simulink model "Airbrake_sim_newpso"  (R2023b)
settings: Solver=FixedStepAuto  StartTime=0.0  StopTime=30  FixedStep=0.01  RelTol=1e-3
model workspace (MAT data in the model file):
  surfaceBlockParameters = Simulink.LookupTable
  surfaceBlockParameters.Table = Simulink.lookuptable.Table
  surfaceBlockParameters.Table.Value = [NaN  NaN  0.380794449822  0.728773534398  NaN  NaN  NaN  NaN  NaN  NaN; NaN  0.340919042573  0.625235126666  0.957009157245  1.00743578256  NaN  NaN  NaN  NaN  NaN; NaN  0.353129064095  0.623587727315  0.932827854759  1.01999161645  0.993209674944  1.00919848998  NaN  NaN  NaN; NaN  0.34799438672  0.580016589939  0.85209505132  1.02225906289  1.00597567868  1.02425853382  1.01771474988  NaN  NaN; NaN  0.226861582106  0.376876909549  0.518810490622  0.672066047723  0.848281603015  0.912315034914  1.01860688625  1.01252755561  NaN; NaN  0.126870515097  0.242227811563  0.341343656012  0.440732304946  0.540686733543  0.640877801771  0.74098706081  0.847669712374  0.948242976715; NaN  0.102593547356  0.219184909799  0.320129045968  0.419935690547  0.51983163298  0.619736559855  0.719639536535  0.819499251087  0.920613400955; NaN  0.126373615097  0.242999668086  0.348071164816  0.45356155619  0.558926581829  0.664568268606  0.769792885801  0.875344669256  0.984850905137; NaN  0.145349212594  0.265578858353  0.378257422798  0.491345121826  0.60466079478  0.718042208189  0.830759161789  0.945577376333  NaN; NaN  0.163436148952  0.285848572034  0.404597762166  0.523292314253  0.642106386903  0.760843310233  0.879580868316  0.998645514796  NaN]
  surfaceBlockParameters.Table.Dimensions = [10 10]
  surfaceBlockParameters.Table.DataType = 'auto'
  surfaceBlockParameters.Table.FieldName = 'Table_zData'
  surfaceBlockParameters.Breakpoints(1) = Simulink.lookuptable.Breakpoint
  surfaceBlockParameters.Breakpoints(1).Value = [0.01 0.2 0.39 0.58 0.77 0.96 1.15 1.34 1.53 1.72]
  surfaceBlockParameters.Breakpoints(1).TunableSizeName = 'N1'
  surfaceBlockParameters.Breakpoints(1).Dimensions = [1 10]
  surfaceBlockParameters.Breakpoints(1).DataType = 'auto'
  surfaceBlockParameters.Breakpoints(1).FieldName = 'BP1_xData'
  surfaceBlockParameters.Breakpoints(2) = Simulink.lookuptable.Breakpoint
  surfaceBlockParameters.Breakpoints(2).Value = [0.33 0.55 0.77 0.99 1.21 1.43 1.65 1.87 2.09 2.31]
  surfaceBlockParameters.Breakpoints(2).TunableSizeName = 'N2'
  surfaceBlockParameters.Breakpoints(2).Dimensions = [1 10]
  surfaceBlockParameters.Breakpoints(2).DataType = 'auto'
  surfaceBlockParameters.Breakpoints(2).FieldName = 'BP2_yData'
  surfaceBlockParameters.AllowMultipleInstancesOfTypeToHaveDifferentTableBreakpointSizes = 0
  surfaceBlockParameters.SupportTunableSize = 0
  surfaceBlockParameters.StructTypeInfo = Simulink.lookuptable.StructTypeInfo
  surfaceBlockParameters.StructTypeInfo.Name = 'surfaceBlockParameters_type'
  surfaceBlockParameters.StructTypeInfo.DataScope = 'Auto'
undefined symbols (not defined in the file or in its folder): apogee, D, dy_mat, I, N, P, t2a, y
libraries: simulink x1, slpidlib x1, shared3dof x1
settings Model: Creator=ruotsing  LastModifiedBy=ruotsing

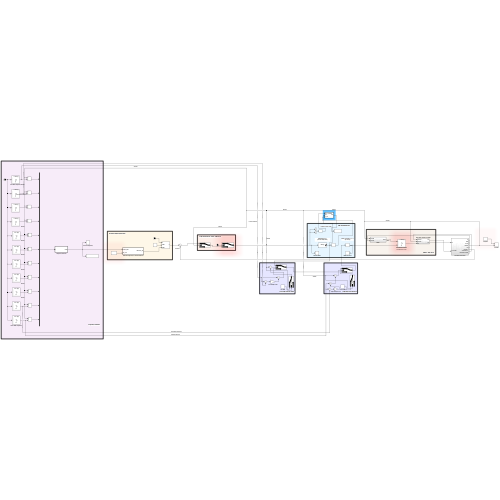
[thumbnail: Simulink's stored preview of the top-level diagram]
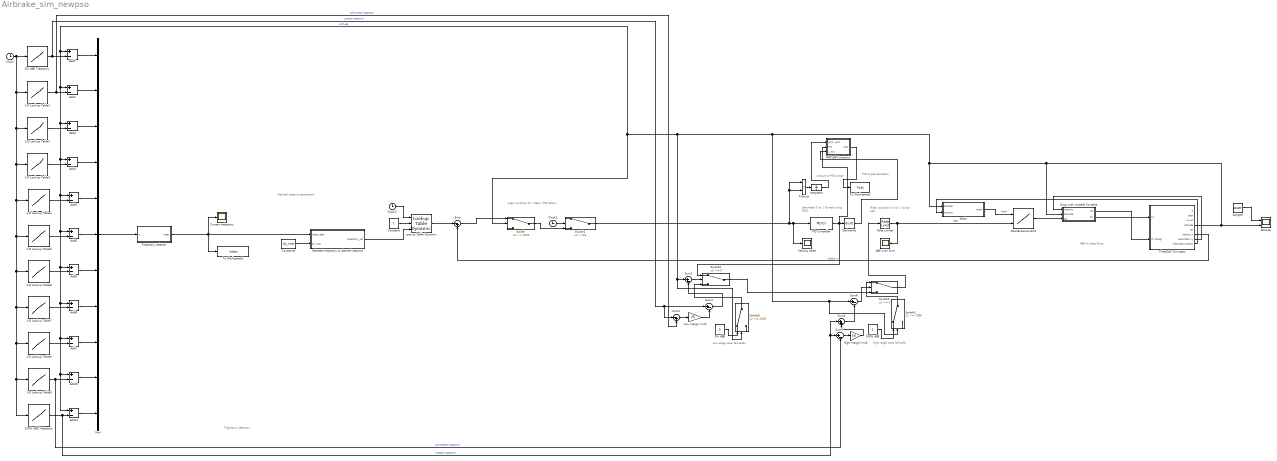
== system Airbrake_sim_newpso ==
  note: ABE to drag force
  note: Trajectory selection
  note: Desired setpoint generation
  note: PID Implementation
  note: Logic switches for "clean" PID action
  note: output to PSO script
  note: Rate constraint -1 to 1
      | (to be set)
  note: Saturated 0 to 1
      | (tuned using PSO)
  note: High edge case fail-safe
  note: Low edge case fail-safes
  0% ABE : Constant  Value=0
  0% ABE Trajectory : Lookup_n-D  NumberOfTableDimensions=1  BreakpointsForDimension1=y{1}.Time  Table=y{1}.Data  InternalRulePriority=Speed  RndMeth=Simplest
  1-D Lookup Table1 : Lookup_n-D  NumberOfTableDimensions=1  BreakpointsForDimension1=y{2}.Time  Table=y{2}.Data  InternalRulePriority=Speed  RndMeth=Simplest
  1-D Lookup Table2 : Lookup_n-D  NumberOfTableDimensions=1  BreakpointsForDimension1=y{3}.Time  Table=y{3}.Data  InternalRulePriority=Speed  RndMeth=Simplest
  1-D Lookup Table3 : Lookup_n-D  NumberOfTableDimensions=1  BreakpointsForDimension1=y{4}.Time  Table=y{4}.Data  InternalRulePriority=Speed  RndMeth=Simplest
  1-D Lookup Table4 : Lookup_n-D  NumberOfTableDimensions=1  BreakpointsForDimension1=y{5}.Time  Table=y{5}.Data  InternalRulePriority=Speed  RndMeth=Simplest
  1-D Lookup Table5 : Lookup_n-D  NumberOfTableDimensions=1  BreakpointsForDimension1=y{6}.Time  Table=y{6}.Data  InternalRulePriority=Speed  RndMeth=Simplest
  1-D Lookup Table6 : Lookup_n-D  NumberOfTableDimensions=1  BreakpointsForDimension1=y{9}.Time  Table=y{9}.Data  InternalRulePriority=Speed  RndMeth=Simplest
  1-D Lookup Table7 : Lookup_n-D  NumberOfTableDimensions=1  BreakpointsForDimension1=y{8}.Time  Table=y{8}.Data  InternalRulePriority=Speed  RndMeth=Simplest
  1-D Lookup Table8 : Lookup_n-D  NumberOfTableDimensions=1  BreakpointsForDimension1=y{7}.Time  Table=y{7}.Data  InternalRulePriority=Speed  RndMeth=Simplest
  1-D Lookup Table9 : Lookup_n-D  NumberOfTableDimensions=1  BreakpointsForDimension1=y{10}.Time  Table=y{10}.Data  InternalRulePriority=Speed  RndMeth=Simplest
  100% ABE : Constant
  100% ABE Trajectory : Lookup_n-D  NumberOfTableDimensions=1  BreakpointsForDimension1=y{11}.Time  Table=y{11}.Data  InternalRulePriority=Speed  RndMeth=Simplest
  ABE over time : Scope
  Add{1..11} (11 alike) : Sum  Inputs=+-
  Altitude : Scope  NumInputPorts=2
  Apogee : Constant  Value=apogee
  Clock : Clock
  Clock1 : Clock
  Clock2 : Clock
  Constant : Constant  Value=t
  Constant3 : Constant  Value=dy_mat  SampleTime=0
  Current trajectory : Scope
  Derivative : Derivative
  Drag with variable Cd table : Subsystem
  High margin mult : Gain  Gain=50
  Integrator : Integrator
  Lookup Table Dynamic : simulink/Lookup Tables/Lookup Table Dynamic  LookUpMeth=Interpolation-Use End Values  OutDataType=fixdt('double')  OutScaling=[]  OutputDataTypeScalingMode=Specify via dialog  OutDataTypeStr=double  DoSatur=off
  Low margin mult : Gain  Gain=25
  MATLAB Function1 : MATLAB Function  TreatAsAtomicUnit=on
  Mach : Subsystem
  MachExtension2Cd : Lookup_n-D  DataSpecification=Lookup table object  LookupTableObject=surfaceBlockParameters1  BreakpointsForDimension1=[1:3]  BreakpointsForDimension2=[1:3]  ExtrapMethod=Clip  InternalRulePriority=Speed  RndMeth=Simplest
      settings: AttributesFormatString=Extrapolation=%<ExtrapMethod>  InputPortMap=u0,u1
  Mux : Mux  Inputs=11
  PID Controller : slpidlib/PID Controller  Controller=PID  Form=Parallel  TimeDomain=Continuous-time  UseExternalTs=off  SampleTime=-1  IntegratorMethod=Forward Euler  FilterMethod=Forward Euler  ControllerParametersSource=internal  P=P  I=I  UseKiTs=off  D=D  N=N  UseFilter=on  TunerSelectOption=Transfer Function Based (PID Tuner App)  InitialConditionSource=internal  InitialConditionForIntegrator=0  InitialConditionForFilter=0  DifferentiatorICPrevScaledInput=0  ExternalReset=none  TrackingMode=off  Kt=1  LimitOutput=on  SatLimitsSource=internal  UpperSaturationLimit=1  LowerSaturationLimit=0  LinearizeAsGain=off  AntiWindupMode=none  Kb=1  LimitIntegrator=off  UpperIntegratorSaturationLimit=inf  LowerIntegratorSaturationLimit=-inf  POutMin=[]  POutMax=[]  IOutMin=[]  IOutMax=[]  DOutMin=[]  DOutMax=[]  NOutMin=[]  NOutMax=[]  SumOutMin=[]  SumOutMax=[]  SaturationOutMin=[]  SaturationOutMax=[]  PParamMin=[]  PParamMax=[]  IParamMin=[]  IParamMax=[]  DParamMin=[]  DParamMax=[]  NParamMin=[]  NParamMax=[]  KbParamMin=[]  KbParamMax=[]  KtParamMin=[]  KtParamMax=[]  KbOutMin=[]  KbOutMax=[]  KtOutMin=[]  KtOutMax=[]  IntegratorOutMin=[]  IntegratorOutMax=[]  FilterOutMin=[]  FilterOutMax=[]  SumI1OutMin=[]  SumI1OutMax=[]  SumI2OutMin=[]  SumI2OutMax=[]  SumI3OutMin=[]  SumI3OutMax=[]  SumI4OutMin=[]  SumI4OutMax=[]  SumDOutMin=[]  SumDOutMax=[]  DifferentiatorOutMin=[]  DifferentiatorOutMax=[]  FilterDiffOutCoefMin=[]  FilterDiffOutCoefMax=[]  ReciprocalOutMin=[]  ReciprocalOutMax=[]  SumDenOutMin=[]  SumDenOutMax=[]  SumNumOutMin=[]  SumNumOutMax=[]  DivideOutMin=[]  DivideOutMax=[]  UdiffTsProdOutMin=[]  UdiffTsProdOutMax=[]  NTsProdOutMin=[]  NTsProdOutMax=[]  UintegralTsProdOutMin=[]  UintegralTsProdOutMax=[]  UngainTsProdOutMin=[]  UngainTsProdOutMax=[]  ClampingZeroOutDataTypeStr=Inherit: Inherit via back propagation  ClampingZeroOutMin=[]  ClampingZeroOutMax=[]  FilterDenConstantOutDataTypeStr=Inherit: Inherit via back propagation  FilterDenConstantOutMin=[]  FilterDenConstantOutMax=[]  PCopyOutDataTypeStr=Inherit: Inherit via back propagation  PCopyOutMin=[]  PCopyOutMax=[]  NCopyOutDataTypeStr=Inherit: Inherit via back propagation  NCopyOutMin=[]  NCopyOutMax=[]  IntegratorContinuousStateAttributes=''  IntegratorStateMustResolveToSignalObject=off  IntegratorRTWStateStorageClass=Auto  FilterContinuousStateAttributes=''  FilterStateMustResolveToSignalObject=off  FilterRTWStateStorageClass=Auto  ParallelPVariant=InternalParameters  IdealPVariant=Disabled  IVariant=InternalParameters  DVariant=InternalParameters  IntegratorVariant=Continuous  SatVariant=Enabled  AWVariant=Passthrough  PCopyVariant=Disabled  TRVariant=Disabled  FdbkBlocksVariant=Forward  IdealPFdbkVariant=Disabled  SatFdbkVariant=Disabled  DerivativeFilterVariant=ContFilter  NVariant=InternalParameters  NCopyVariant=Disabled  FilterICVariant=InternalICsFilter  IntegratorICVariant=InternalICs  ExternalResetVariant=Disabled  TRSumVariant=Passthrough  SumFdbkVariant=Disabled  SumVariant=Sum_PID  TsampFilterVariant=InternalTs  TsampNgainVariant=Passthrough  TsampIntegralVariant=Disabled_SignalSpec  ExternalSaturationOutDataTypeStr=Inherit: Same as second input
  Product : Product
  Rate Limiter : RateLimiter  SampleTimeMode=inherited
  Selected trajectory to desired setpoint : MATLAB Function  TreatAsAtomicUnit=on
  Sum : Sum  Inputs=|-+
  Sum{1,4..6} (4 alike) : Sum  Inputs=|+-
  Sum2 : Sum  Inputs=|-+
  Sum3 : Sum  Inputs=|++
  Switch : Switch  Threshold=2000  SaturateOnIntegerOverflow=off  InputSameDT=off
  Switch1 : Switch  Criteria=u2 > Threshold  Threshold=t2a  SaturateOnIntegerOverflow=off  InputSameDT=off
  Switch2 : Switch  SaturateOnIntegerOverflow=off  InputSameDT=off
  Switch3 : Switch  Threshold=2000  SaturateOnIntegerOverflow=off  InputSameDT=off
  Switch4 : Switch  SaturateOnIntegerOverflow=off  InputSameDT=off
  Switch5 : Switch  Threshold=2000  SaturateOnIntegerOverflow=off  InputSameDT=off
  ThreeDoF Simulator : Subsystem
  To Workspace1 : ToWorkspace  VariableName=Fobj  SampleTime=-1
      settings: Save2DSignal=2-D array (concatenate along first dimension)
  To Workspace2 : ToWorkspace  VariableName=index  SaveFormat=Structure With Time  SampleTime=-1
  Trajectory selector : MATLAB Function  TreatAsAtomicUnit=on
  Velocity delta : Scope
  wires:
  Add1/1 -> Mux/1
  1-D Lookup Table1/1 -> Add2/2, Sum2/2  "2nd lowest trajectory"
  Add2/1 -> Mux/2
  1-D Lookup Table2/1 -> Add3/2
  Add4/1 -> Mux/4
  1-D Lookup Table3/1 -> Add4/2
  Add3/1 -> Mux/3
  1-D Lookup Table4/1 -> Add5/2
  Add5/1 -> Mux/5
  1-D Lookup Table5/1 -> Add6/2
  Add6/1 -> Mux/6
  1-D Lookup Table6/1 -> Add7/2
  Add7/1 -> Mux/9
  1-D Lookup Table7/1 -> Add8/2
  Add8/1 -> Mux/8
  1-D Lookup Table8/1 -> Add9/2
  Add9/1 -> Mux/7
  Add10/1 -> Mux/10
  1-D Lookup Table9/1 -> Sum5/2, Add10/2  "2nd highest trajectory"
  Clock/1 -> 1-D Lookup Table5/1, 1-D Lookup Table8/1, 1-D Lookup Table7/1, 1-D Lookup Table6/1, 1-D Lookup Table9/1, 100% ABE Trajectory/1, 1-D Lookup Table4/1, 1-D Lookup Table3/1, 1-D Lookup Table2/1, 1-D Lookup Table1/1, 0% ABE Trajectory/1
  100% ABE Trajectory/1 -> Add11/2, Sum3/1, Sum5/1  "Highest trajectory"
  Add11/1 -> Mux/11
  Mux/1 -> Trajectory selector/1(u)
  0% ABE Trajectory/1 -> Add1/2, Sum2/1, Sum4/1  "Lowest trajectory"
  ThreeDoF Simulator/4(altitude) -> Drag with variable Cd table/2(Altitude), Switch/2, Add3/1, Add4/1, Add5/1, Add6/1, Add9/1, Add8/1, Add7/1, Add10/1, Add11/1, Add2/1, Add1/1, Switch5/2, Sum1/1, Switch3/2, Sum6/1, Mach/1(Altitude), Altitude/2  "altitude"
  ThreeDoF Simulator/6(velocity z) -> Sum/2  "Velocity z"
  Mach/1(mach) -> MachExtension2Cd/1  "Mach"
  ThreeDoF Simulator/7(velocities z-y) -> Drag with variable Cd table/1(Velocity)
  MachExtension2Cd/1 -> Drag with variable Cd table/3(Cd)
  Drag with variable Cd table/1(Dz) -> ThreeDoF Simulator/2(Fz (Drag))
  Selected trajectory to desired setpoint/1(trajectory_vel) -> Lookup Table Dynamic/3
  Constant/1 -> Lookup Table Dynamic/2
  Clock1/1 -> Lookup Table Dynamic/1
  ThreeDoF Simulator/8(velocities module) -> Mach/2(Velocity)
  Constant3/1 -> Selected trajectory to desired setpoint/2(dy_mat)
  Lookup Table Dynamic/1 -> Sum/1
  Rate Limiter/1 -> MachExtension2Cd/2, ABE over time/1  "ABE"
  Drag with variable Cd table/2(Dx) -> ThreeDoF Simulator/1(Fx)
  Trajectory selector/1(index) -> Current trajectory/1, Selected trajectory to desired setpoint/1(index_data), To Workspace2/1
  Product/1 -> Integrator/1
  Apogee/1 -> Altitude/1
  Clock2/1 -> Switch1/2
  Switch/1 -> Switch1/3
  Sum/1 -> Switch/1
  Sum1/1 -> Switch2/2
  Sum4/1 -> Sum1/2
  Switch3/1 -> Switch4/1
  Sum6/1 -> Switch4/2
  Switch4/1 -> Rate Limiter/1
  100% ABE/1 -> Switch3/1
  Low margin mult/1 -> Sum4/2
  Sum2/1 -> Low margin mult/1
  Sum5/1 -> High margin mult/1
  High margin mult/1 -> Sum3/2
  Sum3/1 -> Sum6/2
  Switch1/1 -> Velocity delta/1, PID Controller/1, Product/1, Product/2
  0% ABE/1 -> Switch5/1
  Switch5/1 -> Switch2/3
  Switch2/1 -> Switch4/3
  Integrator/1 -> MATLAB Function1/1(error_integral)
  Derivative/1 -> MATLAB Function1/3(v_ext)
  PID Controller/1 -> MATLAB Function1/2(ext), Derivative/1, Switch2/1
  MATLAB Function1/1(cost) -> To Workspace1/1

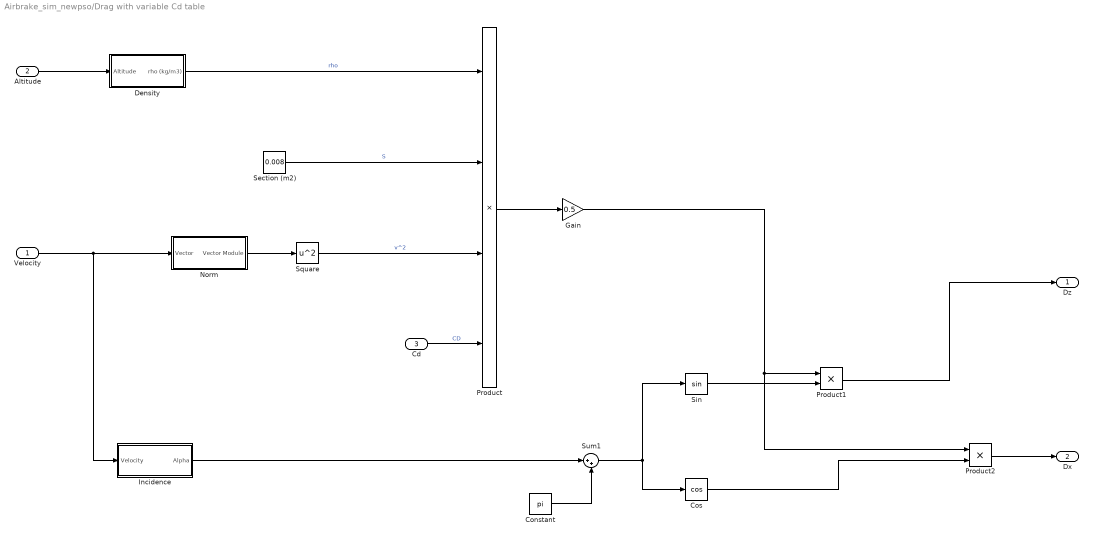
== system Airbrake_sim_newpso/Drag with variable Cd table ==
  Velocity : Inport
  Altitude : Inport  Port=2
  Cd : Inport  Port=3
  Constant : Constant  Value=pi
  Cos : Trigonometry  Operator=cos
  Density : Subsystem
  Gain : Gain  Gain=0.5
  Incidence : Subsystem
  Norm : Subsystem
  Product : Product  Inputs=4
  Product1 : Product
  Product2 : Product
  Section (m2) : Constant  Value=0.008
  Sin : Trigonometry
  Square : Math  Operator=square
  Sum1 : Sum  Inputs=|++
  Dz : Outport
  Dx : Outport  Port=2
  wires:
  Velocity/1 -> Incidence/1(Velocity), Norm/1(Vector)
  Altitude/1 -> Density/1(Altitude)
  Incidence/1(Alpha) -> Sum1/1
  Norm/1(Vector Module) -> Square/1
  Density/1(rho (kg/m3)) -> Product/1  "rho"
  Section (m2)/1 -> Product/2  "S"
  Square/1 -> Product/3  "v^2"
  Product/1 -> Gain/1
  Cd/1 -> Product/4  "CD"
  Constant/1 -> Sum1/2
  Sum1/1 -> Sin/1, Cos/1
  Sin/1 -> Product1/2
  Gain/1 -> Product2/1, Product1/1
  Cos/1 -> Product2/2
  Product2/1 -> Dx/1
  Product1/1 -> Dz/1

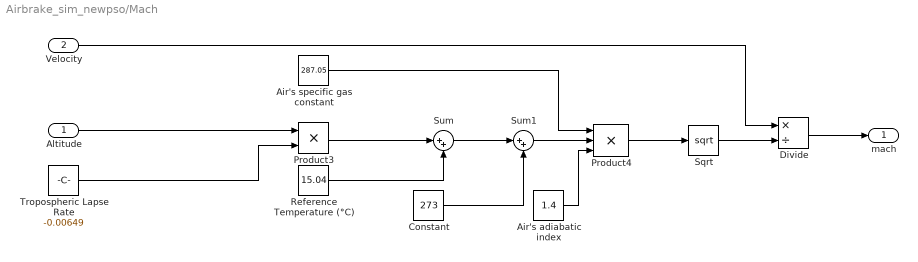
== system Airbrake_sim_newpso/Mach ==
  Altitude : Inport
  Velocity : Inport  Port=2
  Air's adiabatic index : Constant  Value=1.4
  Air's specific gas constant : Constant  Value=287.05
  Constant : Constant  Value=273
  Divide : Product  Inputs=*/
  Product3 : Product
  Product4 : Product  Inputs=3
  Reference Temperature (°C) : Constant  Value=15.04
  Sqrt : Sqrt
  Sum : Sum  Inputs=|++
  Sum1 : Sum  Inputs=|++
  Tropospheric Lapse Rate : Constant  Value=-0.00649
  mach : Outport
  wires:
  Product4/1 -> Sqrt/1
  Product3/1 -> Sum/1
  Air's adiabatic index/1 -> Product4/3
  Tropospheric Lapse Rate/1 -> Product3/2
  Air's specific gas constant/1 -> Product4/1
  Sum/1 -> Sum1/1
  Reference Temperature (°C)/1 -> Sum/2
  Altitude/1 -> Product3/1
  Velocity/1 -> Divide/1
  Divide/1 -> mach/1
  Constant/1 -> Sum1/2
  Sum1/1 -> Product4/2
  Sqrt/1 -> Divide/2

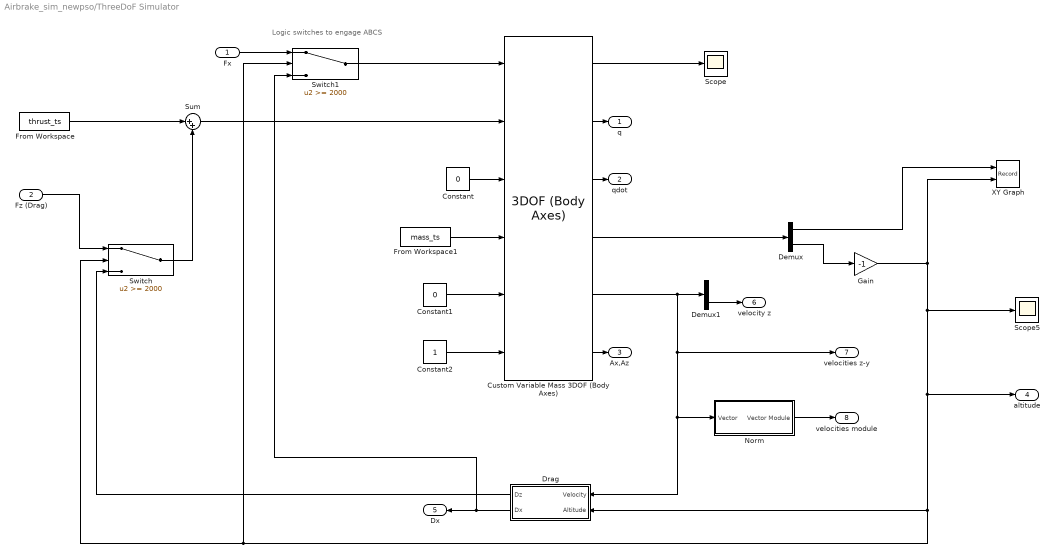
== system Airbrake_sim_newpso/ThreeDoF Simulator ==
  note: Logic switches to engage ABCS
  Fx : Inport
  Fz (Drag) : Inport  Port=2
  Constant : Constant  Value=0
  Constant1 : Constant  Value=0
  Constant2 : Constant
  Custom Variable Mass 3DOF (Body Axes) : shared3dof/3DOF (Body Axes)  units=Metric (MKS)  mtype=Custom Variable  v_ini=0  theta_ini=pi  alpha_ini=0  pos_ini=[0 0]  q_ini=0  mass=1.0  mass_e=0.5  mass_f=3.0  Iyy=1.0  Iyy_e=0.5  Iyy_f=3.0  g_in=Internal  g=9.81  vre_flag=off  abi_flag=off  aMode=0  vel_statename=''  theta_statename=''  pos_statename=''  q_statename=''  mass_statename=''
  Demux : Demux  Outputs=2
  Demux1 : Demux  Outputs=2
  Drag : Subsystem
  From Workspace : FromWorkspace  VariableName=thrust_ts
  From Workspace1 : FromWorkspace  VariableName=mass_ts
  Gain : Gain  Gain=-1
  Norm : Subsystem
  Scope : Scope
  Scope5 : Scope
  Sum : Sum  Inputs=|++
  Switch : Switch  Threshold=2000  SaturateOnIntegerOverflow=off  InputSameDT=off
  Switch1 : Switch  Threshold=2000  SaturateOnIntegerOverflow=off  InputSameDT=off
  XY Graph : Record  FileSettingsInternal="{\"entries\":[{\"content\":{\"excelSettings\":{\"content\":{},\"type\":\"Streamout.ExcelSettings\"}},\"type\":\"Streamout.FileSettingStorage\",\"uuid\":\"\"}],\"packageUris\":[\"http:\\/\\/schema.mathworks.com\\/mf0\\/streamout_blocks\\/R2020a\"],\"version\":\"1.0\"}"  Layout=[1 1]  SignalsInternal="{\"entries\":[{\"content\":{\"signals\":[{\"content\":{\"blockPath\":[],\"dimensions\":[1],\"domain\":\"\",\"lineColor\":\"#0072bd\",\"port\":1,\"signalID\":3349,\"signalName\":\"Demux:1\"},\"type\":\"RecordBlkView.Signal\",\"uuid\":\"\"},{\"content\":{\"blockPath\":[],\"dimensions\":[1],\"domain\":\"\",\"lineColor\":\"#d95319\",\"port\":2,\"signalID\":3352,\"signalName\":\"Gain\"},\"type\":\"RecordBlkView.Signal\",\"uuid\":\"\"}]},\"type\":\"RecordBlkView.InputSignals\",\"uuid\":\"\"}],\"packageUris\":[\"http:\\/\\/schema.mathworks.com\\/mf0\\/streamout_blocks\\/R2020a\"],\"version\":\"1.0\"}"  VisualizationBindings="{\"xyplotplugin\":{\"info\":[{\"series\":[],\"subplotID\":1}]}}"  CompatibilityTag=XY  st=-1
  "q " : Outport
  qdot : Outport  Port=2
  Ax,Az : Outport  Port=3
  altitude : Outport  Port=4
  Dx : Outport  Port=5
  velocity z : Outport  Port=6
  velocities z-y : Outport  Port=7
  velocities module : Outport  Port=8
  wires:
  Constant/1 -> Custom Variable Mass 3DOF (Body Axes)/3
  Custom Variable Mass 3DOF (Body Axes)/6 -> Ax,Az/1
  Demux/2 -> Gain/1
  From Workspace1/1 -> Custom Variable Mass 3DOF (Body Axes)/4
  Custom Variable Mass 3DOF (Body Axes)/2 -> "q "/1
  Demux/1 -> XY Graph/1
  Custom Variable Mass 3DOF (Body Axes)/1 -> Scope/1
  Constant2/1 -> Custom Variable Mass 3DOF (Body Axes)/6
  Constant1/1 -> Custom Variable Mass 3DOF (Body Axes)/5
  Custom Variable Mass 3DOF (Body Axes)/3 -> qdot/1
  Custom Variable Mass 3DOF (Body Axes)/4 -> Demux/1
  Sum/1 -> Custom Variable Mass 3DOF (Body Axes)/2
  Fz (Drag)/1 -> Switch/1
  Gain/1 -> Scope5/1, altitude/1, Drag/2(Altitude), Switch1/2, Switch/2, XY Graph/2
  Drag/2(Dx) -> Switch1/3, Dx/1
  Drag/1(Dz) -> Switch/3
  Switch/1 -> Sum/2
  Demux1/2 -> velocity z/1
  Custom Variable Mass 3DOF (Body Axes)/5 -> Demux1/1, Norm/1(Vector), Drag/1(Velocity), velocities z-y/1
  Norm/1(Vector Module) -> velocities module/1
  Fx/1 -> Switch1/1
  Switch1/1 -> Custom Variable Mass 3DOF (Body Axes)/1
  From Workspace/1 -> Sum/1

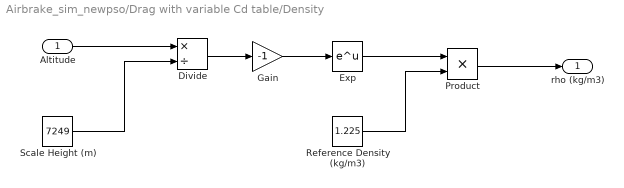
== system Airbrake_sim_newpso/Drag with variable Cd table/Density ==
  Altitude : Inport
  Divide : Product  Inputs=*/
  Exp : Math
  Gain : Gain  Gain=-1
  Product : Product
  Reference Density (kg/m3) : Constant  Value=1.225
  Scale Height (m) : Constant  Value=7249
  rho (kg/m3) : Outport
  wires:
  Altitude/1 -> Divide/1
  Scale Height (m)/1 -> Divide/2
  Divide/1 -> Gain/1
  Gain/1 -> Exp/1
  Exp/1 -> Product/1
  Reference Density (kg/m3)/1 -> Product/2
  Product/1 -> rho (kg/m3)/1

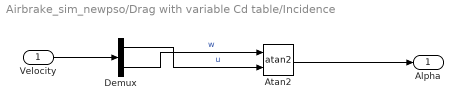
== system Airbrake_sim_newpso/Drag with variable Cd table/Incidence ==
  Velocity : Inport
  Atan2 : Trigonometry  Operator=atan2
  Demux : Demux  Outputs=2
  Alpha : Outport
  wires:
  Velocity/1 -> Demux/1
  Demux/2 -> Atan2/1  "w"
  Demux/1 -> Atan2/2  "u"
  Atan2/1 -> Alpha/1

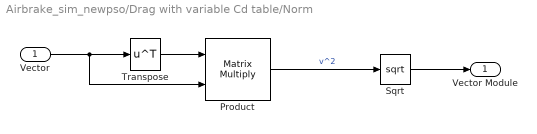
== system Airbrake_sim_newpso/Drag with variable Cd table/Norm ==
  Vector : Inport
  Product : Product  Multiplication=Matrix(*)
  Sqrt : Sqrt
  Transpose : Math  Operator=transpose
  Vector Module : Outport
  wires:
  Vector/1 -> Product/2, Transpose/1
  Product/1 -> Sqrt/1  "v^2"
  Sqrt/1 -> Vector Module/1
  Transpose/1 -> Product/1

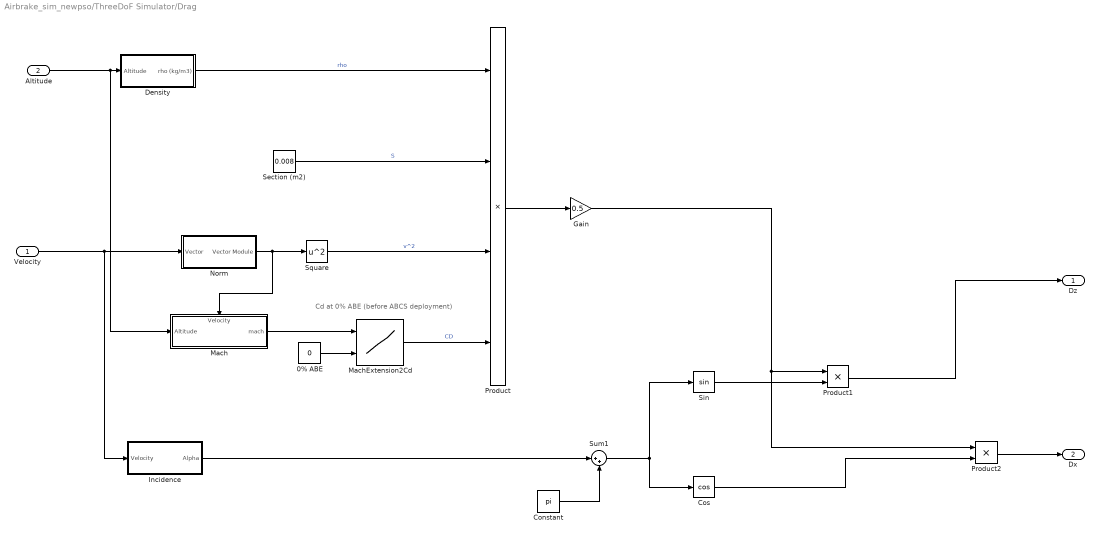
== system Airbrake_sim_newpso/ThreeDoF Simulator/Drag ==
  note: Cd at 0% ABE (before ABCS deployment)
  Velocity : Inport
  Altitude : Inport  Port=2
  0% ABE : Constant  Value=0
  Constant : Constant  Value=pi
  Cos : Trigonometry  Operator=cos
  Density : Subsystem
  Gain : Gain  Gain=0.5
  Incidence : Subsystem
  Mach : Subsystem
      settings: PortSchema="{\"entries\":[{\"content\":{\"sides\":[{\"content\":{\"connectorIds\":[\"In1\"]},\"type\":\"ConnectorPlacement.EquallySpacedRectSide\",\"uuid\":\"3d39723d-d359-4481-8e57-a1560243478f\"},{\"content\":{\"connectorIds\":[\"Out1\"],\"side\":\"RIGHT\"},\"type\":\"ConnectorPlacement.EquallySpacedRectSide\",\"uuid\":\"25d074cf-118b-4153-b466-e753361fe918\"},{\"content\":{\"connectorIds\":[\"In2\"],\"side\":\"TOP\"},\"type\":\"ConnectorPlacement.EquallySpacedRectSide\",\"uuid\":\"b814a212-e79e-4e83-ade8-85d301fd4927\"}]},\"type\":\"ConnectorPlacement.EquallySpacedConnector\",\"uuid\":\"c89f41df-1f7d-46ca-b296-160aff391222\"}],\"packageUris\":[\"http://schema.mathworks.com/mf0/Connector/R2020b\"],\"version\":\"1.0\"}"
  MachExtension2Cd : Lookup_n-D  DataSpecification=Lookup table object  LookupTableObject=surfaceBlockParameters1  BreakpointsForDimension1=[1:3]  BreakpointsForDimension2=[1:3]  ExtrapMethod=Clip  InternalRulePriority=Speed  RndMeth=Simplest
      settings: AttributesFormatString=Extrapolation=%<ExtrapMethod>  InputPortMap=u0,u1
  Norm : Subsystem
  Product : Product  Inputs=4
  Product1 : Product
  Product2 : Product
  Section (m2) : Constant  Value=0.008
  Sin : Trigonometry
  Square : Math  Operator=square
  Sum1 : Sum  Inputs=|++
  Dz : Outport
  Dx : Outport  Port=2
  wires:
  Velocity/1 -> Incidence/1(Velocity), Norm/1(Vector)
  Altitude/1 -> Mach/1(Altitude), Density/1(Altitude)
  Incidence/1(Alpha) -> Sum1/1
  Norm/1(Vector Module) -> Square/1, Mach/2(Velocity)
  Density/1(rho (kg/m3)) -> Product/1  "rho"
  Section (m2)/1 -> Product/2  "S"
  Square/1 -> Product/3  "v^2"
  Product/1 -> Gain/1
  MachExtension2Cd/1 -> Product/4  "CD"
  Constant/1 -> Sum1/2
  Sum1/1 -> Sin/1, Cos/1
  Sin/1 -> Product1/2
  Gain/1 -> Product2/1, Product1/1
  Cos/1 -> Product2/2
  Product2/1 -> Dx/1
  Product1/1 -> Dz/1
  Mach/1(mach) -> MachExtension2Cd/1
  0% ABE/1 -> MachExtension2Cd/2

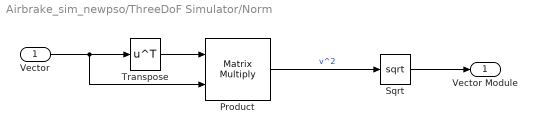
== system Airbrake_sim_newpso/ThreeDoF Simulator/Norm ==
  Vector : Inport
  Product : Product  Multiplication=Matrix(*)
  Sqrt : Sqrt
  Transpose : Math  Operator=transpose
  Vector Module : Outport
  wires:
  Vector/1 -> Product/2, Transpose/1
  Product/1 -> Sqrt/1  "v^2"
  Sqrt/1 -> Vector Module/1
  Transpose/1 -> Product/1

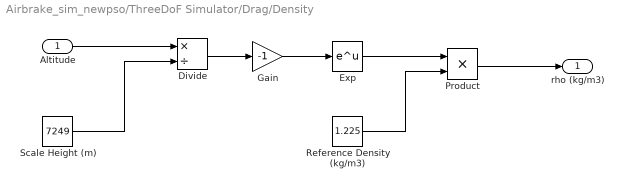
== system Airbrake_sim_newpso/ThreeDoF Simulator/Drag/Density ==
  Altitude : Inport
  Divide : Product  Inputs=*/
  Exp : Math
  Gain : Gain  Gain=-1
  Product : Product
  Reference Density (kg/m3) : Constant  Value=1.225
  Scale Height (m) : Constant  Value=7249
  rho (kg/m3) : Outport
  wires:
  Altitude/1 -> Divide/1
  Scale Height (m)/1 -> Divide/2
  Divide/1 -> Gain/1
  Gain/1 -> Exp/1
  Exp/1 -> Product/1
  Reference Density (kg/m3)/1 -> Product/2
  Product/1 -> rho (kg/m3)/1

== system Airbrake_sim_newpso/ThreeDoF Simulator/Drag/Incidence ==
  Velocity : Inport
  Atan2 : Trigonometry  Operator=atan2
  Demux : Demux  Outputs=2
  Alpha : Outport
  wires:
  Velocity/1 -> Demux/1
  Demux/2 -> Atan2/1  "w"
  Demux/1 -> Atan2/2  "u"
  Atan2/1 -> Alpha/1

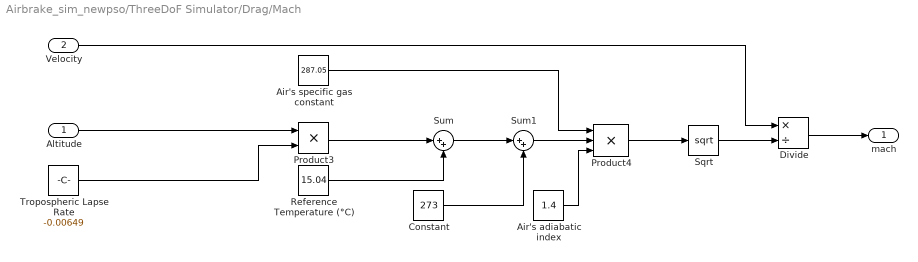
== system Airbrake_sim_newpso/ThreeDoF Simulator/Drag/Mach ==
  Altitude : Inport
  Velocity : Inport  Port=2
  Air's adiabatic index : Constant  Value=1.4
  Air's specific gas constant : Constant  Value=287.05
  Constant : Constant  Value=273
  Divide : Product  Inputs=*/
  Product3 : Product
  Product4 : Product  Inputs=3
  Reference Temperature (°C) : Constant  Value=15.04
  Sqrt : Sqrt
  Sum : Sum  Inputs=|++
  Sum1 : Sum  Inputs=|++
  Tropospheric Lapse Rate : Constant  Value=-0.00649
  mach : Outport
  wires:
  Product4/1 -> Sqrt/1
  Product3/1 -> Sum/1
  Air's adiabatic index/1 -> Product4/3
  Tropospheric Lapse Rate/1 -> Product3/2
  Air's specific gas constant/1 -> Product4/1
  Sum/1 -> Sum1/1
  Reference Temperature (°C)/1 -> Sum/2
  Altitude/1 -> Product3/1
  Velocity/1 -> Divide/1
  Divide/1 -> mach/1
  Constant/1 -> Sum1/2
  Sum1/1 -> Product4/2
  Sqrt/1 -> Divide/2

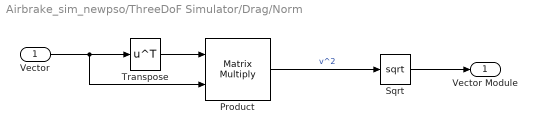
== system Airbrake_sim_newpso/ThreeDoF Simulator/Drag/Norm ==
  Vector : Inport
  Product : Product  Multiplication=Matrix(*)
  Sqrt : Sqrt
  Transpose : Math  Operator=transpose
  Vector Module : Outport
  wires:
  Vector/1 -> Product/2, Transpose/1
  Product/1 -> Sqrt/1  "v^2"
  Sqrt/1 -> Vector Module/1
  Transpose/1 -> Product/1

== matlab function Airbrake_sim_newpso/Selected trajectory to desired setpoint ==
  data: index_data input; trajectory_vel output; dy_mat input
function trajectory_vel = index2traj_vel(index_data,dy_mat)
trajectory_vel = dy_mat(:,index_data);

== matlab function Airbrake_sim_newpso/MATLAB Function1 ==
  data: error_integral input; cost output; ext input; v_ext input
function cost = fcn(error_integral,ext,v_ext)
if ext >1 || ext<0
    cost=inf
end
rate=0.1
cost=0.5*(v_ext-rate)^2+0.5*error_integral

== matlab function Airbrake_sim_newpso/Trajectory selector ==
  data: u input; index output
function index = traj_selector(u)
    
    min_difference = Inf;
    index_of_closest = 0;

    
    for i = 1:length(u)
        
        difference = abs(u(i) - 0);
        
        if difference < min_difference
            
            min_difference = difference;
            index_of_closest = i;
        end
    end
    
    index = index_of_closest;
end
